simulink model "sistema_control_ph"  (R2018a)
settings: Solver=VariableStepAuto  StartTime=0.0  StopTime=100  RelTol=1e-3
InitFcn:
  | sistema_ph
values from neighbouring files (symbols this model uses):
  ki = kt(1,3)    [control_nolineal_linealizacion_entrada_estado.m]    (also in e_mimo.m; ej_mimo.m = kt(:,2+1:end); ej_mimo2.m = kt(:,2+1:end); ejemplo_2.m)
  kp = kt(1,1:2)    [control_nolineal_linealizacion_entrada_estado.m]    (also in e_mimo.m; ej_mimo.m = kt(:,1:2); ej_mimo2.m = kt(:,1:2); ejemplo_2.m)
libraries: simulink x1
settings Model: Creator=carma  LastModifiedBy=carma

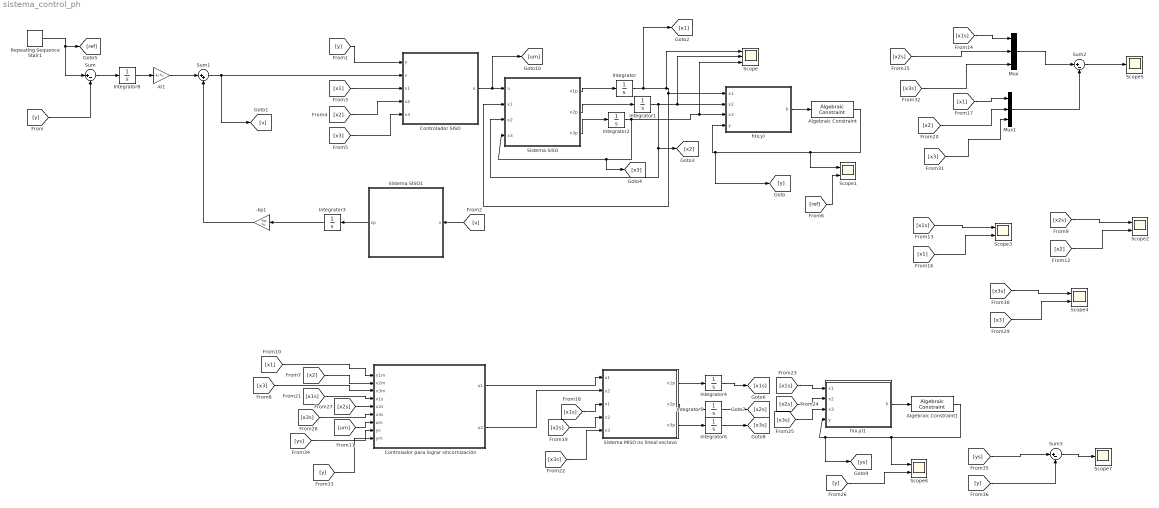
== system sistema_control_ph ==
  -ki1 : Gain  Gain=-ki  Multiplication=Matrix(K*u) (u vector)
  -kp1 : Gain  Gain=-kp  Multiplication=Matrix(K*u) (u vector)
  Algebraic Constraint : AlgebraicConstraint
  Algebraic Constraint1 : AlgebraicConstraint
  Controlador SISO : MATLAB Function  TreatAsAtomicUnit=on
  Controlador para lograr sincornización : MATLAB Function  TreatAsAtomicUnit=on
  Integrator{,1..6,8} (8 alike) : Integrator
  Mux : Mux  Inputs=3
  Mux1 : Mux  Inputs=3
  Repeating Sequence Stair1 : simulink/Sources/Repeating Sequence Stair  OutValues=[9 8 7 6 5 6 7 8].'  tsamp=10  OutMin=[]  OutMax=[]  OutDataTypeStr=double  OutputDataTypeScalingMode=double  OutDataType=fixdt(0,8)  ConRadixGroup=Best Precision: Vector-wise  OutScaling=2^-12
  Scope : Scope  NumInputPorts=3
  Scope{1..4,6} (5 alike) : Scope  NumInputPorts=2
  Scope5 : Scope
  Scope7 : Scope
  Sistema MISO no lineal esclavo : MATLAB Function  TreatAsAtomicUnit=on
  Sistema SISO : MATLAB Function  TreatAsAtomicUnit=on
  Sistema SISO1 : MATLAB Function  TreatAsAtomicUnit=on
  Sum : Sum  Inputs=|+-
  Sum1 : Sum  Inputs=|++
  Sum2 : Sum  Inputs=|+-
  Sum3 : Sum  Inputs=|+-
  h(x,y) : MATLAB Function  TreatAsAtomicUnit=on
  h(x,y)1 : MATLAB Function  TreatAsAtomicUnit=on
  wires:
  Sistema SISO/1(x1p) -> Integrator/1
  Sistema SISO/2(x2p) -> Integrator1/1
  Sistema SISO/3(x3p) -> Integrator2/1
  Integrator2/1 -> Scope/3, h(x,y)/3(x3), [x3], Sistema SISO/4(x3)
  Integrator1/1 -> Scope/2, h(x,y)/2(x2), [x2], Sistema SISO/3(x2)
  Integrator/1 -> [x1], Scope/1, h(x,y)/1(x1), Sistema SISO/2(x1)
  Controlador SISO/1(u) -> [um], Sistema SISO/1(u)
  Sum/1 -> Integrator8/1
  Repeating Sequence Stair1/1 -> [ref], Sum/1
  [y] -> Sum/2
  h(x,y)/1(h) -> Algebraic Constraint/1
  Sistema SISO1/1(zp) -> Integrator3/1
  Integrator3/1 -> -kp1/1
  -kp1/1 -> Sum1/2
  [y] -> Controlador SISO/1(y)
  Integrator8/1 -> -ki1/1
  -ki1/1 -> Sum1/1
  [v] -> Sistema SISO1/1(v)
  Sum1/1 -> [v], Controlador SISO/2(v)
  Algebraic Constraint/1 -> Scope1/1, [y], h(x,y)/4(y)
  [x1] -> Controlador SISO/3(x1)
  [x2] -> Controlador SISO/4(x2)
  [x3] -> Controlador SISO/5(x3)
  [ref] -> Scope1/2
  [x2] -> Mux1/2
  [x2s] -> Scope2/1
  Integrator5/1 -> [x2s]
  [x1s] -> Mux/1
  [x2s] -> Sistema MISO no lineal esclavo/4(x2)
  Mux1/1 -> Sum2/2
  Sistema MISO no lineal esclavo/1(x1p) -> Integrator4/1
  [x1s] -> Sistema MISO no lineal esclavo/3(x1)
  Integrator4/1 -> [x1s]
  Mux/1 -> Sum2/1
  Controlador para lograr sincornización/1(u1) -> Sistema MISO no lineal esclavo/1(u1)
  Sistema MISO no lineal esclavo/2(x2p) -> Integrator5/1
  [x1] -> Scope3/2
  Controlador para lograr sincornización/2(u2) -> Sistema MISO no lineal esclavo/2(u2)
  [x1] -> Controlador para lograr sincornización/1(x1m)
  [x1] -> Mux1/1
  Sum2/1 -> Scope5/1
  [x2] -> Scope2/2
  [x2s] -> Mux/2
  [x1s] -> Scope3/1
  [x2] -> Controlador para lograr sincornización/2(x2m)
  [x3] -> Controlador para lograr sincornización/3(x3m)
  Integrator6/1 -> [x3s]
  Sistema MISO no lineal esclavo/3(x3p) -> Integrator6/1
  [x3s] -> Sistema MISO no lineal esclavo/5(x3)
  [x3s] -> h(x,y)1/3(x3)
  [x2s] -> h(x,y)1/2(x2)
  [x1s] -> h(x,y)1/1(x1)
  h(x,y)1/1(h) -> Algebraic Constraint1/1
  Algebraic Constraint1/1 -> Scope6/1, [ys], h(x,y)1/4(y)
  [x1s] -> Controlador para lograr sincornización/4(x1s)
  [x2s] -> Controlador para lograr sincornización/5(x2s)
  [x3s] -> Controlador para lograr sincornización/6(x3s)
  [um] -> Controlador para lograr sincornización/7(um)
  [y] -> Scope6/2
  [x3s] -> Scope4/1
  [x3] -> Scope4/2
  [x3] -> Mux1/3
  [x3s] -> Mux/3
  [y] -> Controlador para lograr sincornización/9(ym)
  [ys] -> Controlador para lograr sincornización/8(ys)
  [ys] -> Sum3/1
  [y] -> Sum3/2
  Sum3/1 -> Scope7/1

== matlab function sistema_control_ph/Controlador SISO ==
  data: u output; y input; v input; x1 input; x2 input; x3 input
function u = fcn(y,v,x1,x2,x3)

%parametros
V=2900;
a1=0;
a2=0.00305;
a3=5e-5;
c1=0.0255;
c2=0.0255;
w11=0;
w12=3e-3;
w13=0.6;
w21=0;
w22=0.03;
w23=0.03;
q1=16.6;
q2=0.55;
Ka1=4.47e-7;
Ka2=5.62e-11;
pk1=-log10(Ka1);
pk2=-log10(Ka2);
pkw=16.6;
eta=0.05;

% Kc=c1+c2;
% Ki=c1*c2+eta^2;
% v=Kc*e+Ki*ei;
Cx3=(2+10^(pk2-y))/(1+10^(pk2-y)+10^(pk1+pk2-2*y));
%hy=

% Lgy=-10^(-y)+10^(y-pkw)+a1-a2+Cx3*a3;
% Lfy=((q1+q2)*(-10^(-y)+10^(y-pkw))+q1*w11+q2*w21-q1*w12-q2*w22+q1*w13*Cx3+q2*w23*Cx3)*Lgy;%/(hy*V);
% 
% u=(v-Lfy)/(Lgy);



Lgy=(a2 - x2)/(V*(1/10^y*log(10) + 10^(y - pkw)*log(10) - (10^(pk2 - y)*x3*log(10))/(10^(pk2 - y) + 10^(pk1 + pk2 - 2*y) + 1) + (x3*(10^(pk2 - y) + 2)*(2*10^(pk1 + pk2 - 2*y)*log(10) + 10^(pk2 - y)*log(10)))/(10^(pk2 - y) + 10^(pk1 + pk2 - 2*y) + 1)^2)) - (a1 - x1)/(V*(1/10^y*log(10) + 10^(y - pkw)*log(10) - (10^(pk2 - y)*x3*log(10))/(10^(pk2 - y) + 10^(pk1 + pk2 - 2*y) + 1) + (x3*(10^(pk2 - y) + 2)*(2*10^(pk1 + pk2 - 2*y)*log(10) + 10^(pk2 - y)*log(10)))/(10^(pk2 - y) + 10^(pk1 + pk2 - 2*y) + 1)^2)) - ((10^(conj(pk2) - conj(y)) + 2)*(a3 - x3))/(V*(10^(conj(pk1) + conj(pk2) - 2*conj(y)) + 10^(conj(pk2) - conj(y)) + 1)*(1/10^y*log(10) + 10^(y - pkw)*log(10) - (10^(pk2 - y)*x3*log(10))/(10^(pk2 - y) + 10^(pk1 + pk2 - 2*y) + 1) + (x3*(10^(pk2 - y) + 2)*(2*10^(pk1 + pk2 - 2*y)*log(10) + 10^(pk2 - y)*log(10)))/(10^(pk2 - y) + 10^(pk1 + pk2 - 2*y) + 1)^2));
Lfy=((q1*(w12 - x2))/V + (q2*(w22 - x2))/V)/(1/10^y*log(10) + 10^(y - pkw)*log(10) - (10^(pk2 - y)*x3*log(10))/(10^(pk2 - y) + 10^(pk1 + pk2 - 2*y) + 1) + (x3*(10^(pk2 - y) + 2)*(2*10^(pk1 + pk2 - 2*y)*log(10) + 10^(pk2 - y)*log(10)))/(10^(pk2 - y) + 10^(pk1 + pk2 - 2*y) + 1)^2) - ((q1*(w11 - x1))/V + (q2*(w21 - x1))/V)/(1/10^y*log(10) + 10^(y - pkw)*log(10) - (10^(pk2 - y)*x3*log(10))/(10^(pk2 - y) + 10^(pk1 + pk2 - 2*y) + 1) + (x3*(10^(pk2 - y) + 2)*(2*10^(pk1 + pk2 - 2*y)*log(10) + 10^(pk2 - y)*log(10)))/(10^(pk2 - y) + 10^(pk1 + pk2 - 2*y) + 1)^2) - ((10^(conj(pk2) - conj(y)) + 2)*((q1*(w13 - x3))/V + (q2*(w23 - x3))/V))/((10^(conj(pk1) + conj(pk2) - 2*conj(y)) + 10^(conj(pk2) - conj(y)) + 1)*(1/10^y*log(10) + 10^(y - pkw)*log(10) - (10^(pk2 - y)*x3*log(10))/(10^(pk2 - y) + 10^(pk1 + pk2 - 2*y) + 1) + (x3*(10^(pk2 - y) + 2)*(2*10^(pk1 + pk2 - 2*y)*log(10) + 10^(pk2 - y)*log(10)))/(10^(pk2 - y) + 10^(pk1 + pk2 - 2*y) + 1)^2));
u=(v-Lfy)/(Lgy);

== matlab function sistema_control_ph/Sistema SISO ==
  data: u input; x1p output; x1 input; x2 input; x3 input; x2p output; x3p output
function [x1p,x2p,x3p]= fcn(u,x1,x2,x3)

%parametros
V=2900;
a1=0;
a2=0.00305;
a3=5e-5;
%c1=0.0255;
%c2=0.0255;
w11=0;
w12=3e-3;
w13=0.6;
w21=0;
w22=0.03;
w23=0.03;
q1=16.6;
q2=0.55;
Ka1=4.47e-7;
Ka2=5.62e-11;
pk1=-log10(Ka1);
pk2=-log10(Ka2);
pkw=16.6;
%eta=0.05;

x1p=(q1/V)*(w11-x1)+(q2/V)*(w21-x1)+u*(a1-x1)/V;
x2p=(q1/V)*(w12-x2)+(q2/V)*(w22-x2)+u*(a2-x2)/V;
x3p=(q1/V)*(w13-x3)+(q2/V)*(w23-x3)+u*(a3-x3)/V;

%s=5;
%syms y
%Cx3=(2+10^(pk2-y))/(1+10^(pk2-y)+10^(pk1+pk2-2*y));
%h=-x1+x2-x3*Cx3+10^(-y)-10^(y-pkw)==0;

%s=double(solve(h));

== matlab function sistema_control_ph/h(x,y) ==
  data: x1 input; h output; x2 input; x3 input; y input
function h = fcn(x1,x2,x3,y)
Ka1=4.47e-7;
Ka2=5.62e-11;
pk1=-log10(Ka1);
pk2=-log10(Ka2);
pkw=16.6;
Cx3=(2+10^(pk2-y))/(1+10^(pk2-y)+10^(pk1+pk2-2*y));
h=-x1+x2-x3*Cx3+10^(-y)-10^(y-pkw);

== matlab function sistema_control_ph/Controlador para lograr sincornización ==
  data: x1m input; u1 output; x2m input; x3m input; x1s input; x2s input; x3s input; u2 output; um input; ys input; ym input
function [u1,u2] = fcn(x1m,x2m,x3m,x1s,x2s,x3s,um,ys,ym)


%parametros
V=2900;
a1=0;
a2=0.00305;
a3=5e-5;
c1=0.0255;
c2=0.0255;
w11=0;
w12=3e-3;
w13=0.6;
w21=0;
w22=0.03;
w23=0.03;
q1=16.6;
q2=0.55;
Ka1=4.47e-7;
Ka2=5.62e-11;
pk1=-log10(Ka1);
pk2=-log10(Ka2);
pkw=16.6;
eta=0.05;

% Kc=c1+c2;
% Ki=c1*c2+eta^2;
% v=Kc*e+Ki*ei;
% Cx3=(2+10^(pk2-y))/(1+10^(pk2-y)+10^(pk1+pk2-2*y));
% %hy=
% 
% % Lgy=-10^(-y)+10^(y-pkw)+a1-a2+Cx3*a3;
% % Lfy=((q1+q2)*(-10^(-y)+10^(y-pkw))+q1*w11+q2*w21-q1*w12-q2*w22+q1*w13*Cx3+q2*w23*Cx3)*Lgy;%/(hy*V);
% %
% % u=(v-Lfy)/(Lgy);
% 
% 
% 
% Lg1y=(a2 - x2)/(V*(1/10^y*log(10) + 10^(y - pkw)*log(10))) - (a1 - x1)/(V*(1/10^y*log(10) + 10^(y - pkw)*log(10))) - (conj(Cx3)*(a3 - x3))/(V*(1/10^y*log(10) + 10^(y - pkw)*log(10)));
% 
% Lg2y=(w12 - x2)/(V*(1/10^y*log(10) + 10^(y - pkw)*log(10))) - (w11 - x1)/(V*(1/10^y*log(10) + 10^(y - pkw)*log(10))) - (conj(Cx3)*(w13 - x3))/(V*(1/10^y*log(10) + 10^(y - pkw)*log(10)));
% 
% Lfy=(q2*(w22 - x2))/(V*(1/10^y*log(10) + 10^(y - pkw)*log(10))) - (q2*(w21 - x1))/(V*(1/10^y*log(10) + 10^(y - pkw)*log(10))) - (q2*conj(Cx3)*(w23 - x3))/(V*(1/10^y*log(10) + 10^(y - pkw)*log(10)));


k11=1-q2/V;
k22=k11;
k33=k11;
k44=2;

g1=[(a1-x1s)/V;
    (a2-x2s)/V;
    (a3-x3s)/V];


g2=[(w11-x1s)/V;
    (w12-x2s)/V;
    (w13-x3s)/V];

g=[g1 g2];

% g=[g1 g2; 0 0];


f1=(q2/V)*[w21-x1s;
    w22-x2s;
    w23-x3s];

% F=f1-[(q1/V)*(w11-x1m)+(um/V)*(a1-x1m);
%        (q1/V)*(w12-x2m)+(um/V)*(a2-x2m);
%        (q1/V)*(w13-x2m)+(um/V)*(a3-x3m)];
%    
   
F=-[(q1/V)*(w11-x1m)+(um/V)*(a1-x1m);
       (q1/V)*(w12-x2m)+(um/V)*(a2-x2m);
       (q1/V)*(w13-x2m)+(um/V)*(a3-x3m)];

% f1=(q2/V)*[w21-x1s;
%     w22-x2s;
%     w23-x3s;
%     0];
% 
% F=f1-[(q1/V)*(w11-x1m)+(um/V)*(a1-x1m);
%        (q1/V)*(w12-x2m)+(um/V)*(a2-x2m);
%        (q1/V)*(w13-x2m)+(um/V)*(a3-x3m);
%        0];

ex1=x1s-x1m;
ex2=x2s-x2m;
ex3=x3s-x3m;
ey=ys-ym;

v1=-k11*ex1;
v2=-k22*ex2;
v3=-k33*ex3;
v4=-k44*ey;

% v=[v1 v2 v3 v4]';
v=[v1 v2 v3]';


u=pinv(g)*(v-F);

u1=u(1,1);
u2=u(2,1);
% u1=(v-Lfy)/(Lg1y);
% u2=(v-Lfy)/(Lg2y);

== matlab function sistema_control_ph/Sistema SISO1 ==
  data: v input; zp output
function zp = fcn(v)

%parametros
V=2900;
a1=0;
a2=0.00305;
a3=5e-5;
%c1=0.0255;
%c2=0.0255;
w11=0;
w12=3e-3;
w13=0.6;
w21=0;
w22=0.03;
w23=0.03;
q1=16.6;
q2=0.55;
Ka1=4.47e-7;
Ka2=5.62e-11;
pk1=-log10(Ka1);
pk2=-log10(Ka2);
pkw=16.6;
%eta=0.05;

zp=v;

%s=5;
%syms y
%Cx3=(2+10^(pk2-y))/(1+10^(pk2-y)+10^(pk1+pk2-2*y));
%h=-x1+x2-x3*Cx3+10^(-y)-10^(y-pkw)==0;

%s=double(solve(h));

== matlab function sistema_control_ph/Sistema MISO no lineal esclavo ==
  data: u1 input; u2 input; x1 input; x2 input; x1p output; x2p output; x3 input; x3p output
function [x1p,x2p,x3p]= fcn(u1,u2,x1,x2,x3)


%parametros
V=2900;
a1=0;
a2=0.00305;
a3=5e-5;
%c1=0.0255;
%c2=0.0255;
w11=0;
w12=3e-3;
w13=0.6;
w21=0;
w22=0.03;
w23=0.03;
q1=16.6;
q2=0.55;
Ka1=4.47e-7;
Ka2=5.62e-11;
pk1=-log10(Ka1);
pk2=-log10(Ka2);
pkw=16.6;
%eta=0.05;

x1p=(u2/V)*(w11-x1)+(q2/V)*(w21-x1)+u1*(a1-x1)/V;
x2p=(u2/V)*(w12-x2)+(q2/V)*(w22-x2)+u1*(a2-x2)/V;
x3p=(u2/V)*(w13-x3)+(q2/V)*(w23-x3)+u1*(a3-x3)/V;

== matlab function sistema_control_ph/h(x,y)1 ==
  data: x1 input; h output; x2 input; x3 input; y input
function h = fcn(x1,x2,x3,y)
Ka1=4.47e-7;
Ka2=5.62e-11;
pk1=-log10(Ka1);
pk2=-log10(Ka2);
pkw=16.6;
Cx3=(2+10^(pk2-y))/(1+10^(pk2-y)+10^(pk1+pk2-2*y));
h=-x1+x2-x3*Cx3+10^(-y)-10^(y-pkw);
